simulink library "aerospace_common"  (R2022b)
settings: Solver=VariableStepAuto  StartTime=0.0  StopTime=10.0  RelTol=1e-3
values from neighbouring files (symbols this model uses):
  mass = 38    [load_init_states.m]
  momentInertia = [3.46,0,-0.28;0,10,0;-0.28,0,13]    [load_init_states.m]
  RefArea = 0.576    [load_mdl_data.m]
  RefLen = 0.18    [load_mdl_data.m]
  RefSpan = 3.2    [load_mdl_data.m]
  V0 = 40    [load_init_states.m]    (also in trim_lon_HV.m = vGrid(i,j))
libraries: matrix_library x1
settings Model: Creator=matt  LastModifiedBy=matt

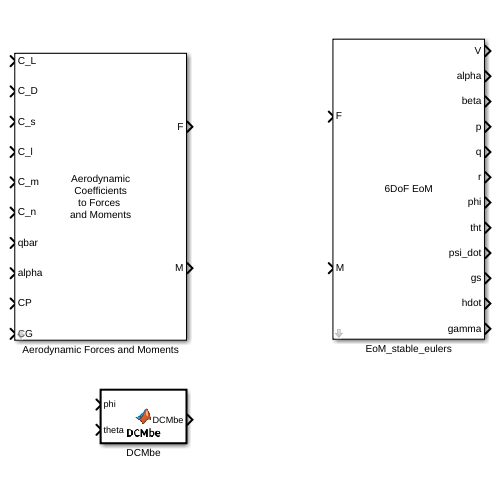
[thumbnail: Simulink's stored preview of the top-level diagram]
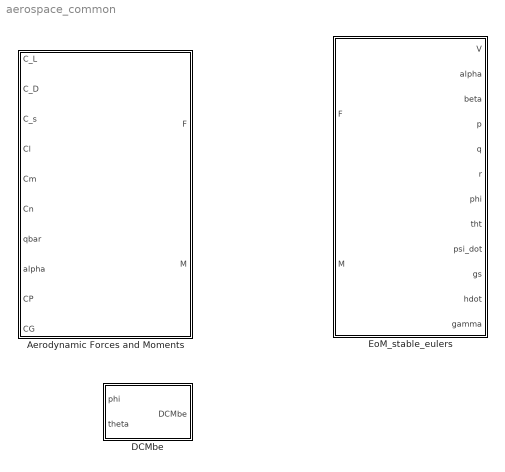
== system aerospace_common ==
  Aerodynamic Forces and Moments : Subsystem  mask{RefArea=RefArea, RefLen=RefLen, RefSpan=RefSpan}
      mask prompts: RefArea "Ref Area"; RefLen "Ref Length"; RefSpan "Ref Span"
      mask Display:
      | disp('Aerodynamic\nCoefficients\nto Forces \nand Moments');
      | port_label('output', 1, 'F');
      | port_label('output', 2, 'M');
      | 
      | port_label('input', 1, 'C_L');
      | port_label('input', 2, 'C_D');
      | port_label('input', 3, 'C_s');
      | port_label('input', 4, 'C_l');
      | port_label('input', 5, 'C_m');
      | port_label('input', 6, 'C_n');
      | port_label('input', 7, 'qbar');
      | port_label('input', 8, 'alpha');
      | port_label('input', 9, 'CP');
      | port_label('input', 10, 'CG');
  DCMbe : MATLAB Function  TreatAsAtomicUnit=on
  EoM_stable_eulers : Subsystem  mask{mass=mass, momentInertia=momentInertia, p0=0, q0=0, r0=0, V0=V0, alpha0=0.03, beta0=0, phi0=0, tht0=0, Parameter11=0}
      mask prompts: p0 "p"; q0 "q"; r0 "r"; V0 "V"; alpha0 "alpha"; beta0 "beta"; phi0 "phi"; tht0 "tht"
      mask DialogControl parameters Prompt: parameters
      mask Display:
      | disp('6DoF EoM');
      | port_label('output', 1, 'V');
      | port_label('output', 2, 'alpha');
      | port_label('output', 3, 'beta');
      | port_label('output', 4, 'p');
      | port_label('output', 5, 'q');
      | port_label('output', 6, 'r');
      | port_label('output', 7, 'phi');
      | port_label('output', 8, 'tht');
      | port_label('output', 9, 'psi_dot');
      | port_label('output', 10, 'gs');
      | port_label('output', 11, 'hdot');
      | port_label('output', 12, 'gamma');
      | port_label('input', 1, 'F');
      | port_label('input', 2, 'M');

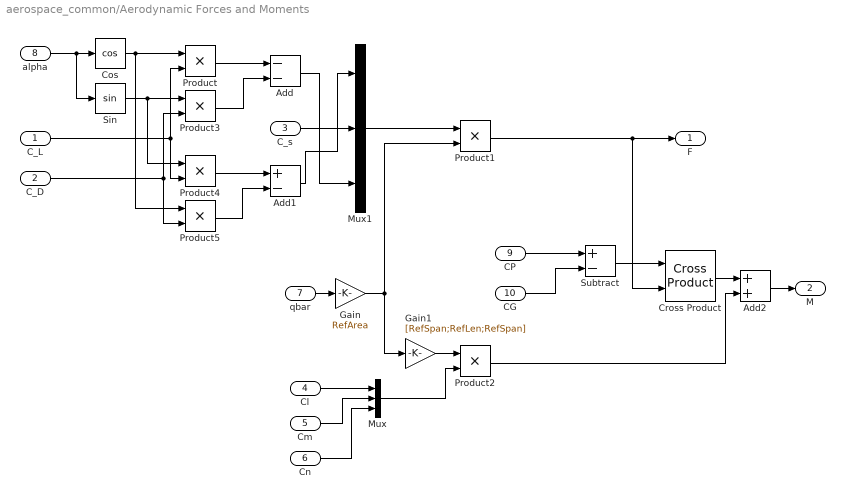
== system aerospace_common/Aerodynamic Forces and Moments ==
  C_L : Inport
  C_D : Inport  Port=2
  C_s : Inport  Port=3
  Cl : Inport  Port=4
  Cm : Inport  Port=5
  Cn : Inport  Port=6
  qbar : Inport  Port=7
  alpha : Inport  Port=8
  CP : Inport  Port=9
  CG : Inport  Port=10
  Add : Sum  Inputs=--
  Add1 : Sum  Inputs=+-
  Add2 : Sum
  Cos : Trigonometry  Operator=cos
  Cross Product : matrix_library/Cross Product
  Gain : Gain  Gain=RefArea
  Gain1 : Gain  Gain=[RefSpan;RefLen;RefSpan]
  Mux : Mux  Inputs=3
  Mux1 : Mux  Inputs=3
  Product{,1..5} (6 alike) : Product
  Sin : Trigonometry
  Subtract : Sum  Inputs=+-
  F : Outport  PortDimensions=[3 1]
  M : Outport  Port=2  PortDimensions=[3 1]
  wires:
  qbar/1 -> Gain/1
  Gain/1 -> Product1/2, Gain1/1
  Product1/1 -> Cross Product/2, F/1
  Product2/1 -> Add2/2
  Gain1/1 -> Product2/1
  Cl/1 -> Mux/1
  Cm/1 -> Mux/2
  Cn/1 -> Mux/3
  Mux/1 -> Product2/2
  alpha/1 -> Sin/1, Cos/1
  C_L/1 -> Product4/2, Product/2
  Sin/1 -> Product4/1, Product3/1
  C_D/1 -> Product5/2, Product3/2
  Product/1 -> Add/1
  Product3/1 -> Add/2
  Cos/1 -> Product5/1, Product/1
  Product4/1 -> Add1/1
  Product5/1 -> Add1/2
  Add/1 -> Mux1/3
  C_s/1 -> Mux1/2
  Add1/1 -> Mux1/1
  Mux1/1 -> Product1/1
  CP/1 -> Subtract/1
  CG/1 -> Subtract/2
  Subtract/1 -> Cross Product/1
  Cross Product/1 -> Add2/1
  Add2/1 -> M/1

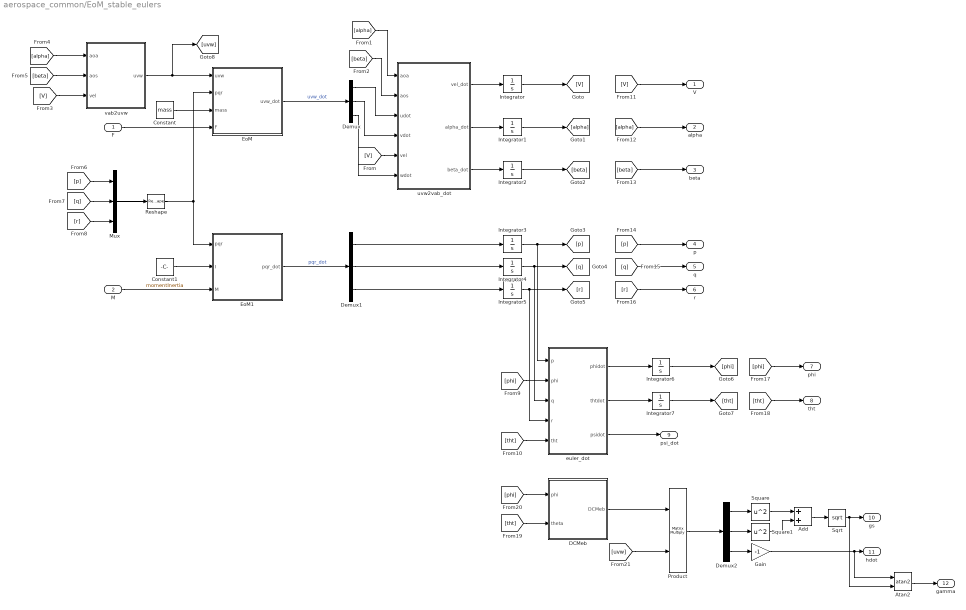
== system aerospace_common/EoM_stable_eulers ==
  F : Inport  PortDimensions=[3,1]
  M : Inport  Port=2  PortDimensions=[3 1]
  Add : Sum
  Atan2 : Trigonometry  Operator=atan2
  Constant : Constant  Value=mass
  Constant1 : Constant  Value=momentInertia
  DCMeb : MATLAB Function  TreatAsAtomicUnit=on
  Demux : Demux  Outputs=3
  Demux1 : Demux  Outputs=3
  Demux2 : Demux  Outputs=3
  EoM : MATLAB Function  TreatAsAtomicUnit=on
  EoM1 : MATLAB Function  TreatAsAtomicUnit=on
  Gain : Gain  Gain=-1
  Integrator : Integrator  InitialCondition=V0  ContinuousStateAttributes='V'
  Integrator1 : Integrator  InitialCondition=alpha0  ContinuousStateAttributes='alpha'
  Integrator2 : Integrator  InitialCondition=beta0  ContinuousStateAttributes='beta'
  Integrator3 : Integrator  InitialCondition=p0  ContinuousStateAttributes='p'
  Integrator4 : Integrator  InitialCondition=q0  ContinuousStateAttributes='q'
  Integrator5 : Integrator  InitialCondition=r0  ContinuousStateAttributes='r'
  Integrator6 : Integrator  InitialCondition=phi0  ContinuousStateAttributes='phi'
  Integrator7 : Integrator  InitialCondition=tht0  ContinuousStateAttributes='tht'
  Mux : Mux  Inputs=3
  Product : Product  Multiplication=Matrix(*)
  Reshape : Reshape  OutputDimensionality=Column vector (2-D)
  Sqrt : Sqrt
  Square : Math  Operator=square
  Square1 : Math  Operator=square
  euler_dot : MATLAB Function  TreatAsAtomicUnit=on
  uvw2vab_dot : MATLAB Function  TreatAsAtomicUnit=on
  vab2uvw : MATLAB Function  TreatAsAtomicUnit=on
  V : Outport
  alpha : Outport  Port=2
  beta : Outport  Port=3
  p : Outport  Port=4
  q : Outport  Port=5
  r : Outport  Port=6
  phi : Outport  Port=7
  tht : Outport  Port=8
  psi_dot : Outport  Port=9
  gs : Outport  Port=10
  hdot : Outport  Port=11
  gamma : Outport  Port=12
  wires:
  [p] -> Mux/1
  [tht] -> euler_dot/5(tht)
  Mux/1 -> Reshape/1
  [tht] -> tht/1
  Demux/3 -> uvw2vab_dot/6(wdot)
  [V] -> uvw2vab_dot/5(vel)
  [beta] -> uvw2vab_dot/2(aos)
  Integrator7/1 -> [tht]
  Integrator6/1 -> [phi]
  Constant/1 -> EoM/3(mass)
  vab2uvw/1(uvw) -> [uvw], EoM/1(uvw)
  [r] -> Mux/3
  Demux/1 -> uvw2vab_dot/3(udot)
  [alpha] -> vab2uvw/1(aoa)
  [V] -> vab2uvw/3(vel)
  [p] -> p/1
  [beta] -> beta/1
  Integrator/1 -> [V]
  [q] -> q/1
  [alpha] -> uvw2vab_dot/1(aoa)
  uvw2vab_dot/2(alpha_dot) -> Integrator1/1
  uvw2vab_dot/1(vel_dot) -> Integrator/1
  [r] -> r/1
  [phi] -> euler_dot/2(phi)
  Demux1/2 -> Integrator4/1
  euler_dot/2(thtdot) -> Integrator7/1
  Integrator1/1 -> [alpha]
  Integrator2/1 -> [beta]
  Demux1/1 -> Integrator3/1
  Integrator3/1 -> euler_dot/1(p), [p]
  [V] -> V/1
  Constant1/1 -> EoM1/2(I)
  M/1 -> EoM1/3(M)
  [beta] -> vab2uvw/2(aos)
  uvw2vab_dot/3(beta_dot) -> Integrator2/1
  euler_dot/3(psidot) -> psi_dot/1
  euler_dot/1(phidot) -> Integrator6/1
  EoM/1(uvw_dot) -> Demux/1  "uvw_dot"
  F/1 -> EoM/4(F)
  Integrator4/1 -> euler_dot/3(q), [q]
  Integrator5/1 -> euler_dot/4(r), [r]
  Demux1/3 -> Integrator5/1
  [phi] -> phi/1
  EoM1/1(pqr_dot) -> Demux1/1  "pqr_dot"
  [q] -> Mux/2
  [alpha] -> alpha/1
  Demux/2 -> uvw2vab_dot/4(vdot)
  Reshape/1 -> EoM1/1(pqr), EoM/2(pqr)
  [phi] -> DCMeb/1(phi)
  [tht] -> DCMeb/2(theta)
  DCMeb/1(DCMeb) -> Product/1
  [uvw] -> Product/2
  Product/1 -> Demux2/1
  Demux2/1 -> Square/1
  Demux2/2 -> Square1/1
  Square/1 -> Add/1
  Square1/1 -> Add/2
  Add/1 -> Sqrt/1
  Sqrt/1 -> Atan2/2, gs/1
  Demux2/3 -> Gain/1
  Gain/1 -> Atan2/1, hdot/1
  Atan2/1 -> gamma/1

== matlab function aerospace_common/EoM_stable_eulers/uvw2vab_dot ==
  data: aoa input; vel_dot output; aos input; udot input; vdot input; vel input; wdot input; alpha_dot output; beta_dot output
function [vel_dot,alpha_dot,beta_dot] = uvw2vab_dot(aoa,aos,udot,vdot,vel,wdot)
%#codegen

%    This function was generated by the Symbolic Math Toolbox version 9.2.
%    02-Dec-2022 13:31:08

t2 = cos(aoa);
t3 = cos(aos);
t4 = sin(aoa);
t5 = sin(aos);
vel_dot = t5.*vdot+t2.*t3.*udot+t3.*t4.*wdot;
if nargout > 1
    t6 = 1.0./vel;
    alpha_dot = -(t6.*(t4.*udot-t2.*wdot))./t3;
end
if nargout > 2
    beta_dot = -t6.*(-t3.*vdot+t2.*t5.*udot+t4.*t5.*wdot);
end

== matlab function aerospace_common/EoM_stable_eulers/EoM ==
  data: uvw input size=[3 1]; uvw_dot output size=[3 1]; pqr input size=[3 1]; mass input size=1; F input size=[3 1]
function uvw_dot = fcn(uvw, pqr, mass, F)

uvw_dot = F/mass - cross(pqr, uvw);

== matlab function aerospace_common/EoM_stable_eulers/vab2uvw ==
  data: uvw output; aoa input; aos input; vel input
function uvw = vab2uvw(aoa,aos,vel)
%#codegen

%    This function was generated by the Symbolic Math Toolbox version 9.2.
%    02-Dec-2022 13:31:08

t2 = cos(aos);
uvw = [t2.*vel.*cos(aoa);vel.*sin(aos);t2.*vel.*sin(aoa)];

== matlab function aerospace_common/EoM_stable_eulers/EoM1 ==
  data: pqr input size=[3 1]; I input size=[3 3]; M input size=[3 1]; pqr_dot output size=[3 1]
function pqr_dot = fcn(pqr, I, M)

pqr_dot = I\(M - cross(pqr, I*pqr));

== matlab function aerospace_common/EoM_stable_eulers/euler_dot ==
  data: p input; phidot output; phi input; q input; r input; tht input; thtdot output; psidot output
function [phidot,thtdot,psidot] = euler_dot(p,phi,q,r,tht)
%#codegen

%    This function was generated by the Symbolic Math Toolbox version 9.2.
%    02-Dec-2022 13:33:09

t2 = cos(phi);
t3 = cos(tht);
t4 = sin(phi);
t5 = sin(tht);
t6 = 1.0./t3;
phidot = t6.*(p.*t3+q.*t4.*t5+r.*t2.*t5);
if nargout > 1
    thtdot = q.*t2-r.*t4;
end
if nargout > 2
    psidot = t6.*(q.*t4+r.*t2);
end

== matlab function aerospace_common/DCMbe ==
  data: phi input; DCMbe output; theta input
function DCMbe = DCMbe(phi,theta)
%#codegen

%    This function was generated by the Symbolic Math Toolbox version 9.2.
%    02-Dec-2022 14:37:26

t2 = cos(phi);
t3 = cos(theta);
t4 = sin(phi);
t5 = sin(theta);
DCMbe = reshape([t3,t4.*t5,t2.*t5,0.0,t2,-t4,-t5,t3.*t4,t2.*t3],[3,3]);

== matlab function aerospace_common/EoM_stable_eulers/DCMeb ==
  data: phi input; DCMeb output; theta input
function DCMeb = DCMeb(phi,theta)
%#codegen

%    This function was generated by the Symbolic Math Toolbox version 9.2.
%    02-Dec-2022 23:22:49

t2 = cos(phi);
t3 = cos(theta);
t4 = sin(phi);
t5 = sin(theta);
DCMeb = reshape([t3,0.0,-t5,t4.*t5,t2,t3.*t4,t2.*t5,-t4,t2.*t3],[3,3]);
